simulink model "Quarter_Car"  (R2019a)
settings: Solver=VariableStepAuto  StartTime=0.0  StopTime=60  RelTol=1e-3
libraries: fl_lib x20, nesl_utility x11, simulink_extras x3, eeGeneralControl x2, sdl_lib x2, simulink x1
settings Model: Creator=Owen Heaney  LastModifiedBy=Owen Heaney

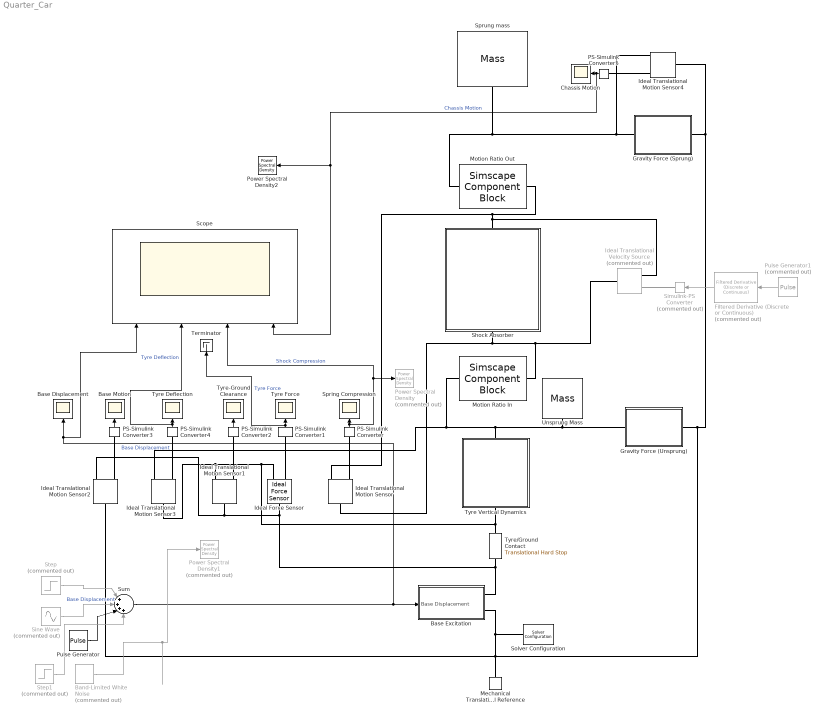
== system Quarter_Car ==
  " Scope" : Scope  NumInputPorts=4
  Band-Limited White Noise : simulink/Sources/Band-Limited White Noise  Commented=on  Cov=[0.5]  Ts=0.1  seed=[23341]
  Base Displacement : Scope
  Base Motion : Scope
  Base Excitation : Subsystem
  Chassis Motion : Scope
  Filtered Derivative (Discrete or Continuous) : eeGeneralControl/Filtered Derivative (Discrete or Continuous)  Commented=on  K=1  T=0.1  B=inf  A=-inf  minRatio=10  Ts=0
      settings: SourceProductName=Simscape Electrical  SourceProductBaseCode=PS
  Gravity Force (Sprung) : Subsystem  mask{m=75}
      mask prompts: m "Mass"
  Gravity Force (Unsprung) : Subsystem  mask{m=5}
      mask prompts: m "Mass"
  Ideal Force Sensor : fl_lib/Mechanical/Mechanical Sensors/Ideal Force Sensor
  Ideal Translational Motion Sensor : fl_lib/Mechanical/Mechanical Sensors/Ideal Translational Motion Sensor  offset=0 mm
  Ideal Translational Motion Sensor{1..4} (4 alike) : fl_lib/Mechanical/Mechanical Sensors/Ideal Translational Motion Sensor  offset=0 m
  Ideal Translational Velocity Source : fl_lib/Mechanical/Mechanical Sources/Ideal Translational Velocity Source  Commented=on
  Mechanical Translational Reference : fl_lib/Mechanical/Translational Elements/Mechanical Translational Reference
  Motion Ratio In : SimscapeComponentBlock  SourceFile=motion_ratio  ComponentPath=motion_ratio  ComponentVariants=motion_ratio  ComponentVariantNames=motion_ratio  ClassName=motion_ratio  SchemaVersion=1  ratio=1.4  f_in_specify=off  f_in_priority=None  f_in=0 N  f_in_nominal_specify=off  f_in_nominal_unit=N  f_in_nominal_value=1  f_out_specify=off  f_out_priority=None  f_out=0 N  f_out_nominal_specify=off  f_out_nominal_unit=N  f_out_nominal_value=1
      settings: CopyFcn=simscape.engine.sli.internal.componentblockcallback(gcbh,'COPY')  PreCopyFcn=simscape.engine.sli.internal.componentblockcallback(gcbh,'PRECOPY')  PreDeleteFcn=simscape.engine.sli.internal.componentblockcallback(gcbh,'PREDELETE')
      mask Type: Motion Ratio
  Motion Ratio Out : SimscapeComponentBlock  SourceFile=motion_ratio  ComponentPath=motion_ratio  ComponentVariants=motion_ratio  ComponentVariantNames=motion_ratio  ClassName=motion_ratio  SchemaVersion=1  ratio=1.4  f_in_specify=off  f_in_priority=None  f_in=0 N  f_in_nominal_specify=off  f_in_nominal_unit=N  f_in_nominal_value=1  f_out_specify=off  f_out_priority=None  f_out=0 N  f_out_nominal_specify=off  f_out_nominal_unit=N  f_out_nominal_value=1
      settings: CopyFcn=simscape.engine.sli.internal.componentblockcallback(gcbh,'COPY')  PreCopyFcn=simscape.engine.sli.internal.componentblockcallback(gcbh,'PRECOPY')  PreDeleteFcn=simscape.engine.sli.internal.componentblockcallback(gcbh,'PREDELETE')
      mask Type: Motion Ratio
  PS-Simulink Converter{,2..5} (5 alike) : nesl_utility/PS-Simulink Converter  PhysicalDomain=network_engine_domain  SubClassName=ps_output  LeftPortType=input  RightPortType=output  PseudoPeriodic=off  Frequencies=[]  Unit=mm  AffineConversion=off
  PS-Simulink Converter1 : nesl_utility/PS-Simulink Converter  PhysicalDomain=network_engine_domain  SubClassName=ps_output  LeftPortType=input  RightPortType=output  PseudoPeriodic=off  Frequencies=[]  Unit=N  AffineConversion=off
  Power Spectral Density : simulink_extras/Additional Sinks/Power Spectral Density  Commented=on  npts=350  fftpts=350  HowOften=350  sampleT=0.1
      settings: SourceProductName=Simulink  SourceProductBaseCode=SL
  Power Spectral Density1 : simulink_extras/Additional Sinks/Power Spectral Density  Commented=on  npts=400  fftpts=400  HowOften=400  sampleT=0.1
      settings: SourceProductName=Simulink  SourceProductBaseCode=SL
  Power Spectral Density2 : simulink_extras/Additional Sinks/Power Spectral Density  npts=128  fftpts=512  HowOften=64  sampleT=0.1
      settings: SourceProductName=Simulink  SourceProductBaseCode=SL
  Pulse Generator : DiscretePulseGenerator  PulseType=Time based  Amplitude=5  Period=10  PulseWidth=50  PhaseDelay=6
  Pulse Generator1 : DiscretePulseGenerator  Commented=on  PulseType=Time based  Amplitude=-1  Period=10  PulseWidth=50  PhaseDelay=6
  Shock Absorber : Subsystem  mask{k=43781.7, F_PL=-1000}
      mask prompts: k "Spring Stiffness"; F_PL "Spring Preload"
      mask Display: image('Shock_Icon.png');
  Simulink-PS Converter : nesl_utility/Simulink-PS Converter  Commented=on  PhysicalDomain=network_engine_domain  SubClassName=ps_input  LeftPortType=input  RightPortType=output  PseudoPeriodic=off  Frequencies=[]  NoiseDistribution=none  NoiseParameters=[]  Unit=mm/s  AffineConversion=off  FilteringAndDerivatives=filter  SimscapeFilterOrder=2  InputFilterTimeConstant=0.001  UdotUserProvided=0
  Sine Wave : Sin  Commented=on  Amplitude=0.1  Frequency=25  SampleTime=0
  Solver Configuration : nesl_utility/Solver Configuration  PhysicalDomain=network_engine_domain  SubClassName=solver  LeftPortType=input  RightPortType=generic  Tones=[]  Harmonics=[]  SimulateNoise=off  Profile=off  UseLocalSampling=off  EnableSwitchedLinearOptims=on  FrequencyDomain=off  UseCCode=off  RelTol=0.001  AbsTol=1e-06  MinStep=1e-09  ToWorkspace=off  RevertToSquareIcSolve=off  NumHomotopyIterations=100  PhasorMode=off  PhasorModeNumHarmonics=1  DoDC=on  ResidualTolerance=1e-15  UseLocalSolver=off  LocalSolverChoice=NE_BACKWARD_EULER_ADVANCER  LocalSolverSampleTime=0.001  DoFixedCost=off  MaxNonlinIter=3  MaxModeIter=2  LinearAlgebra=auto  EquationFormulation=NE_TIME_EF  DelaysMemoryBudget=1024  AutomaticFiltering=on  FilteringTimeConstant=0.001  PartitionStorageMethod=AS_NEEDED  PartitionMemoryBudget=1024  PartitionMethod=ROBUST
  Spring Compression : Scope
  Sprung mass : fl_lib/Mechanical/Translational Elements/Mass  mass=75 kg  v_specify=off  v_priority=High  v=0 m/s  v_nominal_specify=off  v_nominal_unit=m/s  v_nominal_value=1  f_specify=off  f_priority=None  f=0 N  f_nominal_specify=off  f_nominal_unit=N  f_nominal_value=1
  Step : Step  Commented=on  SampleTime=0
  Step1 : Step  Commented=on  After=10  SampleTime=0
  Sum : Sum  Inputs=|++++
  Terminator : Terminator
  Tyre Deflection : Scope
  Tyre Force : Scope
  Tyre Vertical Dynamics : Subsystem  mask{k=80000, m=0.01, c=7}
      mask prompts: k "Tyre Stiffness"; m "Tyre Inertance (Effective mass)"; c "Tyre Damping"
      mask Display: image('Tyre Icon.png');
  Tyre-Ground Clearance : Scope
  Tyre/Ground Contact : fl_lib/Mechanical/Translational Elements/Translational Hard Stop  upper_bnd=100 m  lower_bnd=0 mm  stiff_up=2e6 N/m  stiff_low=2e6 N/m  D_up=150 N/(m/s)  D_low=150 N/(m/s)  model=simscape.enum.hardstop.fulldamped  transition=00.1 mm  v_specify=off  v_priority=None  v=0 m/s  v_nominal_specify=off  v_nominal_unit=m/s  v_nominal_value=1  f_specify=off  f_priority=None  f=0 N  f_nominal_specify=off  f_nominal_unit=N  f_nominal_value=1  x_specify=on  x_priority=High  x=1 m  x_nominal_specify=off  x_nominal_unit=m  x_nominal_value=1
  Unsprung Mass : fl_lib/Mechanical/Translational Elements/Mass  mass=10 kg  v_specify=off  v_priority=High  v=0 m/s  v_nominal_specify=off  v_nominal_unit=m/s  v_nominal_value=1  f_specify=on  f_priority=None  f=-0.01 N  f_nominal_specify=off  f_nominal_unit=N  f_nominal_value=1
  wires:
  PS-Simulink Converter/1 -> Power Spectral Density/1, " Scope"/3, Spring Compression/1  "Shock Compression"
  PS-Simulink Converter1/1 -> Terminator/1, Tyre Force/1  "Tyre Force"
  PS-Simulink Converter2/1 -> Tyre-Ground Clearance/1
  PS-Simulink Converter3/1 -> Base Motion/1
  PS-Simulink Converter4/1 -> " Scope"/2, Tyre Deflection/1  "Tyre Deflection"
  PS-Simulink Converter5/1 -> " Scope"/4, Power Spectral Density2/1, Chassis Motion/1  "Chassis Motion"
  Sine Wave/1 -> Sum/2  "Base Displacement"
  Pulse Generator/1 -> Sum/3
  Sum/1 -> " Scope"/1, Base Displacement/1, Base Excitation/1(Base Displacement)  "Base Displacement"
  Step/1 -> Sum/1
  Band-Limited White Noise/1 -> Power Spectral Density1/1
  Filtered Derivative (Discrete or Continuous)/1 -> Simulink-PS Converter/1
  Pulse Generator1/1 -> Filtered Derivative (Discrete or Continuous)/1
  Step1/1 -> Sum/4
  connections:
  Gravity Force (Sprung)/LConn1 -- Ideal Translational Motion Sensor4/RConn1 -- Motion Ratio Out/LConn1 -- Sprung mass/LConn1
  Ideal Translational Motion Sensor2/LConn1 -- Mechanical Translational Reference/LConn1 -- Gravity Force (Unsprung)/RConn1 -- Ideal Translational Motion Sensor4/LConn1 -- Gravity Force (Sprung)/RConn1 -- Solver Configuration/RConn1 -- Base Excitation/RConn2
  PS-Simulink Converter/LConn1 -- Ideal Translational Motion Sensor/RConn3
  PS-Simulink Converter2/LConn1 -- Ideal Translational Motion Sensor1/RConn3
  PS-Simulink Converter3/LConn1 -- Ideal Translational Motion Sensor2/RConn3
  PS-Simulink Converter4/LConn1 -- Ideal Translational Motion Sensor3/RConn3
  Ideal Force Sensor/RConn1 -- Tyre/Ground Contact/LConn1 -- Tyre Vertical Dynamics/RConn1 -- Ideal Translational Motion Sensor3/LConn1 -- Ideal Translational Motion Sensor1/RConn1
  Unsprung Mass/LConn1 -- Gravity Force (Unsprung)/LConn1 -- Ideal Translational Motion Sensor3/RConn1 -- Motion Ratio In/LConn1 -- Tyre Vertical Dynamics/LConn1
  Ideal Translational Motion Sensor4/RConn3 -- PS-Simulink Converter5/LConn1
  Ideal Force Sensor/RConn2 -- PS-Simulink Converter1/LConn1
  Ideal Force Sensor/LConn1 -- Base Excitation/RConn1 -- Tyre/Ground Contact/RConn1 -- Ideal Translational Motion Sensor1/LConn1 -- Ideal Translational Motion Sensor2/RConn1
  Shock Absorber/LConn1 -- Ideal Translational Velocity Source/RConn2 -- Ideal Translational Motion Sensor/RConn1 -- Motion Ratio Out/RConn1
  Motion Ratio In/RConn1 -- Shock Absorber/RConn1 -- Ideal Translational Motion Sensor/LConn1 -- Ideal Translational Velocity Source/LConn1
  Simulink-PS Converter/RConn1 -- Ideal Translational Velocity Source/RConn1

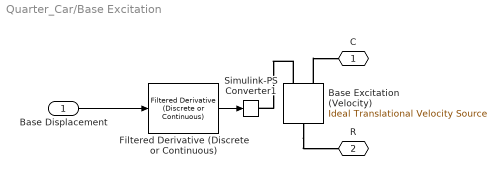
== system Quarter_Car/Base Excitation ==
  Base Displacement : Inport
  Base Excitation (Velocity) : fl_lib/Mechanical/Mechanical Sources/Ideal Translational Velocity Source
  Filtered Derivative (Discrete or Continuous) : eeGeneralControl/Filtered Derivative (Discrete or Continuous)  K=1  T=0.0001  B=inf  A=-inf  minRatio=10  Ts=0
      settings: SourceProductName=Simscape Electrical  SourceProductBaseCode=PS
  Simulink-PS Converter1 : nesl_utility/Simulink-PS Converter  PhysicalDomain=network_engine_domain  SubClassName=ps_input  LeftPortType=input  RightPortType=output  PseudoPeriodic=off  Frequencies=[]  NoiseDistribution=none  NoiseParameters=[]  Unit=mm/s  AffineConversion=off  FilteringAndDerivatives=filter  SimscapeFilterOrder=1  InputFilterTimeConstant=0.001  UdotUserProvided=0
  C : PMIOPort  Side=Right
  R : PMIOPort  Port=2  Side=Right
  wires:
  Base Displacement/1 -> Filtered Derivative (Discrete or Continuous)/1
  Filtered Derivative (Discrete or Continuous)/1 -> Simulink-PS Converter1/1
  connections:
  Base Excitation (Velocity)/RConn1 -- Simulink-PS Converter1/RConn1
  Base Excitation (Velocity)/RConn2 -- C/RConn1
  Base Excitation (Velocity)/LConn1 -- R/RConn1

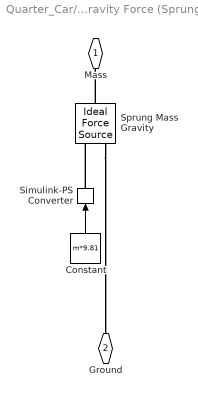
== system Quarter_Car/Gravity Force (Sprung) ==
  Constant : Constant  Value=m*9.81
  Simulink-PS Converter : nesl_utility/Simulink-PS Converter  PhysicalDomain=network_engine_domain  SubClassName=ps_input  LeftPortType=input  RightPortType=output  PseudoPeriodic=off  Frequencies=[]  NoiseDistribution=none  NoiseParameters=[]  Unit=1  AffineConversion=off  FilteringAndDerivatives=provide  SimscapeFilterOrder=1  InputFilterTimeConstant=0.001  UdotUserProvided=0
  Sprung Mass Gravity : fl_lib/Mechanical/Mechanical Sources/Ideal Force Source
  Mass : PMIOPort  Side=Left
  Ground : PMIOPort  Port=2  Side=Right
  wires:
  Constant/1 -> Simulink-PS Converter/1
  connections:
  Simulink-PS Converter/RConn1 -- Sprung Mass Gravity/RConn1
  Sprung Mass Gravity/RConn2 -- Ground/RConn1
  Sprung Mass Gravity/LConn1 -- Mass/RConn1

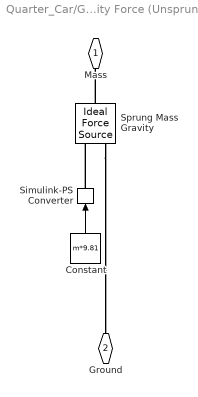
== system Quarter_Car/Gravity Force (Unsprung) ==
  Constant : Constant  Value=m*9.81
  Simulink-PS Converter : nesl_utility/Simulink-PS Converter  PhysicalDomain=network_engine_domain  SubClassName=ps_input  LeftPortType=input  RightPortType=output  PseudoPeriodic=off  Frequencies=[]  NoiseDistribution=none  NoiseParameters=[]  Unit=1  AffineConversion=off  FilteringAndDerivatives=provide  SimscapeFilterOrder=1  InputFilterTimeConstant=0.001  UdotUserProvided=0
  Sprung Mass Gravity : fl_lib/Mechanical/Mechanical Sources/Ideal Force Source
  Mass : PMIOPort  Side=Left
  Ground : PMIOPort  Port=2  Side=Right
  wires:
  Constant/1 -> Simulink-PS Converter/1
  connections:
  Sprung Mass Gravity/LConn1 -- Mass/RConn1
  Sprung Mass Gravity/RConn2 -- Ground/RConn1
  Simulink-PS Converter/RConn1 -- Sprung Mass Gravity/RConn1

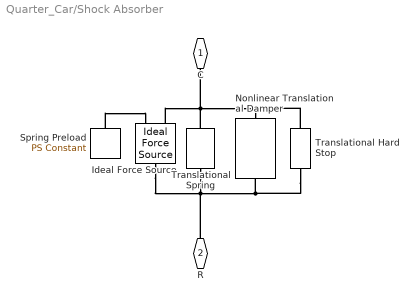
== system Quarter_Car/Shock Absorber ==
  Ideal Force Source : fl_lib/Mechanical/Mechanical Sources/Ideal Force Source
  Nonlinear Translational Damper : sdl_lib/Couplings & Drives/Springs & Dampers/Nonlinear Translational Damper  parameterization=2  symmetry=2  coefficient_vector=[10, 0, 1, 0, .1] N/(m/s)  extension_coefficient_vector=[10, 0, 1, 0, .1] N/(m/s)  contraction_coefficient_vector=[100, -1, 10, 0, 0] N/(m/s)  velocity_vector=[-22.4504384315274,-12.4504384315274,0,11.0953608496650,21.0953608496650] mm/s  force_vector=[-286.421566423866,-280.660930931408,0,299.946509620207,307.630346868698] N  interp_method=simscape.enum.interpolation.linear  extrap_method=simscape.enum.extrapolation.linear
      settings: SourceProductName=Simscape Driveline  SourceProductBaseCode=LD
  Spring Preload : fl_lib/Physical Signals/Sources/PS Constant  constant=F_PL N
  Translational Hard Stop : fl_lib/Mechanical/Translational Elements/Translational Hard Stop  upper_bnd=0 mm  lower_bnd=-57 mm  stiff_up=1e10 N/m  stiff_low=1e10 N/m  D_up=150 N/(m/s)  D_low=150 N/(m/s)  model=simscape.enum.hardstop.smooth  transition=0.1 mm  v_specify=off  v_priority=None  v=0 m/s  v_nominal_specify=off  v_nominal_unit=m/s  v_nominal_value=1  f_specify=off  f_priority=None  f=0 N  f_nominal_specify=off  f_nominal_unit=N  f_nominal_value=1  x_specify=off  x_priority=High  x=0 m  x_nominal_specify=off  x_nominal_unit=m  x_nominal_value=1
  Translational Spring : fl_lib/Mechanical/Translational Elements/Translational Spring  spr_rate=k N/m  v_specify=on  v_priority=High  v=0 m/s  v_nominal_specify=off  v_nominal_unit=m/s  v_nominal_value=1  f_specify=off  f_priority=None  f=0 N  f_nominal_specify=off  f_nominal_unit=N  f_nominal_value=1  x_specify=off  x_priority=High  x=-25 mm  x_nominal_specify=off  x_nominal_unit=m  x_nominal_value=1
  C : PMIOPort  Side=Left
  R : PMIOPort  Port=2  Side=Right
  connections:
  C/RConn1 -- Ideal Force Source/RConn2 -- Translational Spring/RConn1 -- Translational Hard Stop/RConn1 -- Nonlinear Translational Damper/RConn1
  Spring Preload/RConn1 -- Ideal Force Source/RConn1
  R/RConn1 -- Ideal Force Source/LConn1 -- Translational Hard Stop/LConn1 -- Nonlinear Translational Damper/LConn1 -- Translational Spring/LConn1

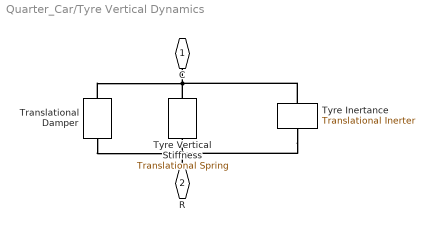
== system Quarter_Car/Tyre Vertical Dynamics ==
  Translational Damper : sdl_lib/Couplings & Drives/Springs & Dampers/Translational Damper  D=c N/(m/s)  enable_faults=0  b_fault=1e6 N/(m/s)  temporal_fault=0  fault_time=5 s  shock_fault=0  acceleration_limit=100 m/s^2  shock_limit=1  report_fault=1
      settings: SourceProductName=Simscape Driveline  SourceProductBaseCode=LD
  Tyre Inertance : fl_lib/Mechanical/Translational Elements/Translational Inerter  B=m kg  v_specify=off  v_priority=High  v=0 m/s  v_nominal_specify=off  v_nominal_unit=m/s  v_nominal_value=1  f_specify=off  f_priority=None  f=0 N  f_nominal_specify=off  f_nominal_unit=N  f_nominal_value=1
      settings: SourceProductName=Simscape  SourceProductBaseCode=SS
  Tyre Vertical Stiffness : fl_lib/Mechanical/Translational Elements/Translational Spring  spr_rate=k N/m  v_specify=on  v_priority=None  v=0 m/s  v_nominal_specify=off  v_nominal_unit=m/s  v_nominal_value=1  f_specify=off  f_priority=None  f=0 N  f_nominal_specify=off  f_nominal_unit=N  f_nominal_value=1  x_specify=off  x_priority=High  x=0 m  x_nominal_specify=off  x_nominal_unit=m  x_nominal_value=1
  C : PMIOPort  Side=Left
  R : PMIOPort  Port=2  Side=Right
  connections:
  Tyre Vertical Stiffness/RConn1 -- Tyre Inertance/RConn1 -- C/RConn1 -- Translational Damper/RConn1
  R/RConn1 -- Tyre Inertance/LConn1 -- Translational Damper/LConn1 -- Tyre Vertical Stiffness/LConn1
